simulink model "SimpleMotorModel"  (R2019b)
settings: Solver=VariableStepAuto  StartTime=0.0  StopTime=0.05  RelTol=1e-3
PreLoadFcn:
  | modelDir = fileparts(get_param(bdroot, 'FileName'));
  | addpath(fullfile(modelDir,'../Parameters'));
  | addpath(fullfile(modelDir,'subsystems'));
  | 
  | Parameters_Model
  | Parameters_Simulation
  | Parameters_Controller
InitFcn:
  | Parameters_Model
  | Parameters_Simulation
  | Parameters_Controller
undefined symbols (not defined in the file): Ke, Ki, Kp, L, R, Ts, w
libraries: cstblocks x2, simulink x1
settings Model: Creator=Thomas  LastModifiedBy=thomas.jespersen
settings DataIOCC: ReturnWorkspaceOutputs=off
settings DebuggingCC: ArithmeticOperatorsInVariantConditions=warning
settings SFSimCC: SimUseLocalCustomCode=off  CustomCodeUndefinedFunction=UseInterfaceOnly
settings RTWCC: RTWUseLocalCustomCode=off

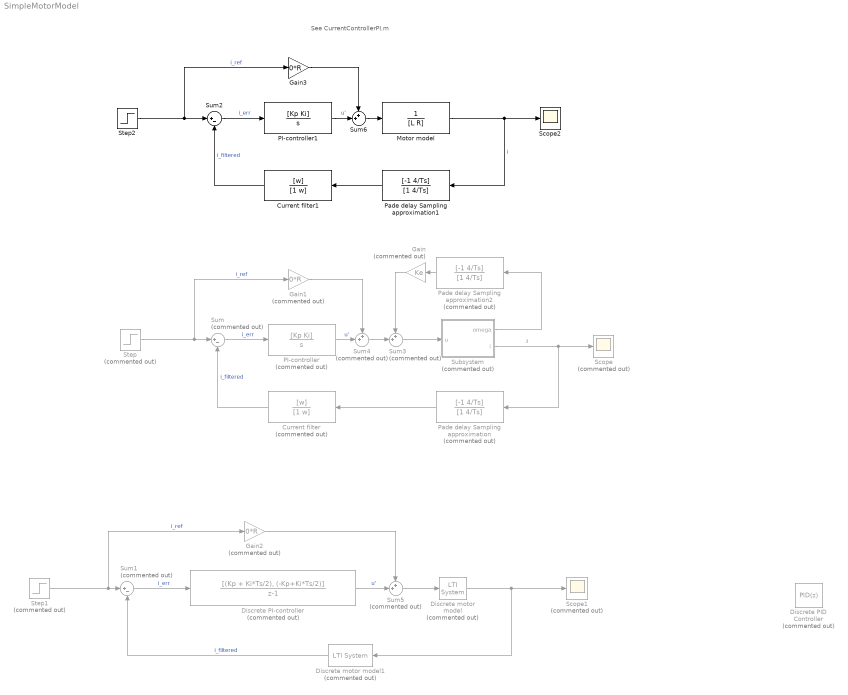
== system SimpleMotorModel ==
  note: See CurrentControllerPI.m
  Current filter : TransferFcn  Commented=on  Numerator=[w]  Denominator=[1 w]
  Current filter1 : TransferFcn  Numerator=[w]  Denominator=[1 w]
  Discrete PI-controller : DiscreteTransferFcn  Commented=on  Numerator=[(Kp + Ki*Ts/2), (-Kp+Ki*Ts/2)]  Denominator=[1 -1]
  Discrete PID Controller : simulink/Continuous/PID Controller  Commented=on  Controller=PID  Form=Parallel  TimeDomain=Discrete-time  SampleTime=-1  IntegratorMethod=Forward Euler  FilterMethod=Forward Euler  ControllerParametersSource=internal  P=1  I=1  D=0  UseFilter=on  N=100  TunerSelectOption=Transfer Function Based (PID Tuner App)  InitialConditionSource=internal  InitialConditionForIntegrator=0  InitialConditionForFilter=0  DifferentiatorICPrevScaledInput=0  ExternalReset=none  TrackingMode=off  Kt=1  LimitOutput=off  UpperSaturationLimit=inf  LowerSaturationLimit=-inf  LinearizeAsGain=off  AntiWindupMode=none  Kb=1  POutMin=[]  POutMax=[]  IOutMin=[]  IOutMax=[]  DOutMin=[]  DOutMax=[]  NOutMin=[]  NOutMax=[]  SumOutMin=[]  SumOutMax=[]  SaturationOutMin=[]  SaturationOutMax=[]  PParamMin=[]  PParamMax=[]  IParamMin=[]  IParamMax=[]  DParamMin=[]  DParamMax=[]  NParamMin=[]  NParamMax=[]  KbParamMin=[]  KbParamMax=[]  KtParamMin=[]  KtParamMax=[]  KbOutMin=[]  KbOutMax=[]  KtOutMin=[]  KtOutMax=[]  IntegratorOutMin=[]  IntegratorOutMax=[]  FilterOutMin=[]  FilterOutMax=[]  SumI1OutMin=[]  SumI1OutMax=[]  SumI2OutMin=[]  SumI2OutMax=[]  SumI3OutMin=[]  SumI3OutMax=[]  SumI4OutMin=[]  SumI4OutMax=[]  SumDOutMin=[]  SumDOutMax=[]  DifferentiatorOutMin=[]  DifferentiatorOutMax=[]  FilterDiffOutCoefMin=[]  FilterDiffOutCoefMax=[]  ReciprocalOutMin=[]  ReciprocalOutMax=[]  SumDenOutMin=[]  SumDenOutMax=[]  SumNumOutMin=[]  SumNumOutMax=[]  DivideOutMin=[]  DivideOutMax=[]  IntegratorContinuousStateAttributes=''  IntegratorStateMustResolveToSignalObject=off  IntegratorRTWStateStorageClass=Auto  FilterContinuousStateAttributes=''  FilterStateMustResolveToSignalObject=off  FilterRTWStateStorageClass=Auto  ParallelPVariant=InternalParameters  IdealPVariant=Disabled  IVariant=InternalParameters  DVariant=InternalParameters  IntegratorVariant=Discrete  SatVariant=Disabled  AWVariant=Passthrough  PCopyVariant=Disabled  TRVariant=Disabled  FdbkBlocksVariant=Forward  IdealPFdbkVariant=Disabled  SatFdbkVariant=Disabled  DerivativeFilterVariant=ForwardEulerFilter  NVariant=InternalParameters  NCopyVariant=Disabled  FilterICVariant=InternalICsFilter  IntegratorICVariant=InternalICs  ExternalResetVariant=Disabled  TRSumVariant=Passthrough  SumFdbkVariant=Disabled  SumVariant=Sum_PID
  Discrete motor model : cstblocks/LTI System  Commented=on  sys=Gd  IC=[]
  Discrete motor model1 : cstblocks/LTI System  Commented=on  sys=Hd_LPF  IC=[]
  Gain : Gain  Commented=on  Gain=Ke
  Gain1 : Gain  Commented=on  Gain=0*R
  Gain2 : Gain  Commented=on  Gain=0*R
  Gain3 : Gain  Gain=0*R
  Motor model : TransferFcn  Denominator=[L R]
  PI-controller : TransferFcn  Commented=on  Numerator=[Kp Ki]  Denominator=[1 0]
  PI-controller1 : TransferFcn  Numerator=[Kp Ki]  Denominator=[1 0]
  Pade delay Sampling approximation : TransferFcn  Commented=on  Numerator=[-1 4/Ts]  Denominator=[1 4/Ts]
  Pade delay Sampling approximation1 : TransferFcn  Numerator=[-1 4/Ts]  Denominator=[1 4/Ts]
  Pade delay Sampling approximation2 : TransferFcn  Commented=on  Numerator=[-1 4/Ts]  Denominator=[1 4/Ts]
  Scope : Scope  Commented=on
  Scope1 : Scope  Commented=on
  Scope2 : Scope
  Step : Step  Commented=on  Time=0.01  SampleTime=0
  Step1 : Step  Commented=on  Time=0.01  SampleTime=0
  Step2 : Step  Time=0.01  SampleTime=0
  Subsystem : Subsystem  Commented=on
  Sum : Sum  Commented=on  Inputs=|+-
  Sum1 : Sum  Commented=on  Inputs=|+-
  Sum2 : Sum  Inputs=|+-
  Sum3 : Sum  Commented=on  Inputs=++|
  Sum4 : Sum  Commented=on  Inputs=++|
  Sum5 : Sum  Commented=on  Inputs=++|
  Sum6 : Sum  Inputs=++|
  wires:
  Current filter/1 -> Sum/2  "i_filtered"
  PI-controller/1 -> Sum4/2  "u'"
  Sum/1 -> PI-controller/1  "i_err"
  Step/1 -> Gain1/1, Sum/1  "i_ref"
  Subsystem/2(i) -> Scope/1, Pade delay Sampling approximation/1  "i"
  Pade delay Sampling approximation/1 -> Current filter/1
  Discrete PI-controller/1 -> Sum5/2  "u'"
  Discrete motor model1/1 -> Sum1/2  "i_filtered"
  Sum1/1 -> Discrete PI-controller/1  "i_err"
  Step1/1 -> Gain2/1, Sum1/1  "i_ref"
  Discrete motor model/1 -> Scope1/1, Discrete motor model1/1
  Motor model/1 -> Scope2/1, Pade delay Sampling approximation1/1  "i"
  Current filter1/1 -> Sum2/2  "i_filtered"
  Pade delay Sampling approximation1/1 -> Current filter1/1
  Sum2/1 -> PI-controller1/1  "i_err"
  PI-controller1/1 -> Sum6/2  "u'"
  Subsystem/1(omega) -> Pade delay Sampling approximation2/1
  Pade delay Sampling approximation2/1 -> Gain/1
  Sum3/1 -> Subsystem/1(u)
  Gain/1 -> Sum3/1
  Sum4/1 -> Sum3/2
  Gain1/1 -> Sum4/1
  Sum5/1 -> Discrete motor model/1
  Gain2/1 -> Sum5/1
  Step2/1 -> Gain3/1, Sum2/1  "i_ref"
  Gain3/1 -> Sum6/1
  Sum6/1 -> Motor model/1

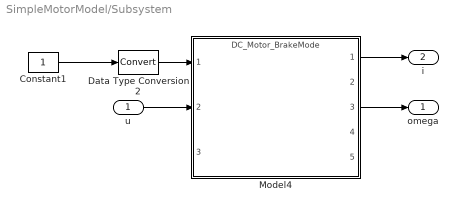
== system SimpleMotorModel/Subsystem ==
  u : Inport
  Constant1 : Constant
  Data Type Conversion2 : DataTypeConversion  RndMeth=Round
  Model4 : ModelReference  ModelNameDialog=DC_Motor_BrakeMode  SimulationMode=Normal  ModelReferenceVersion=1.46
  omega : Outport  VectorParamsAs1DForOutWhenUnconnected=off
  i : Outport  Port=2  VectorParamsAs1DForOutWhenUnconnected=off
  wires:
  Constant1/1 -> Data Type Conversion2/1
  Model4/1 -> i/1
  Data Type Conversion2/1 -> Model4/1
  u/1 -> Model4/2
  Model4/3 -> omega/1
